simulink model "spring_mass"  (R2021b)
settings: Solver=VariableStepAuto  StartTime=0.0  StopTime=10.0  RelTol=1e-3
settings Model: Creator=cgrundm  LastModifiedBy=cgrundm

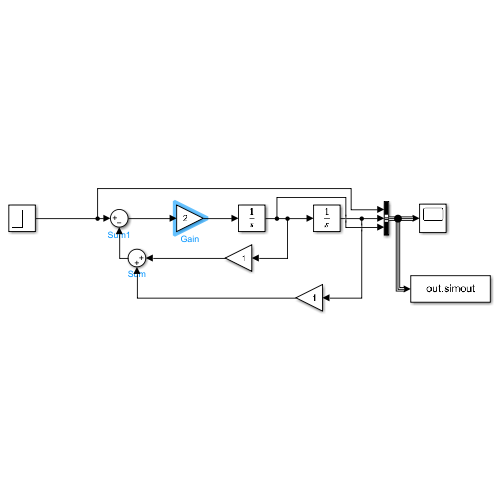
[thumbnail: Simulink's stored preview of the top-level diagram]
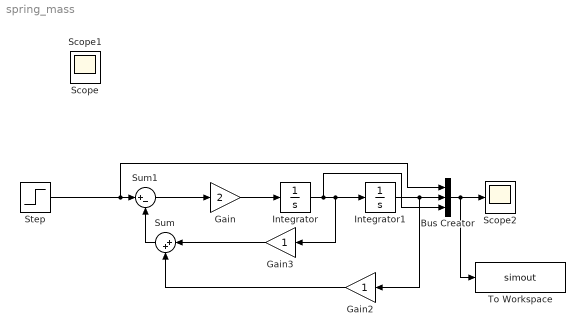
== system spring_mass ==
  Bus Creator : BusCreator  Inputs=3
  Gain : Gain  Gain=2
  Gain2 : Gain
  Gain3 : Gain
  Integrator : Integrator
  Integrator1 : Integrator
  Scope2 : Scope
  Step : Step  SampleTime=0
  Sum : Sum  Inputs=|++
  Sum1 : Sum  Inputs=|+-
  To Workspace : ToWorkspace  VariableName=simout  SaveFormat=Timeseries  SampleTime=-1
  Scope : Scope
  Scope1 : Scope
  wires:
  Integrator1/1 -> Gain2/1, Bus Creator/2
  Integrator/1 -> Bus Creator/3, Gain3/1, Integrator1/1
  Gain3/1 -> Sum/1
  Gain2/1 -> Sum/2
  Step/1 -> Bus Creator/1, Sum1/1
  Sum/1 -> Sum1/2
  Sum1/1 -> Gain/1
  Gain/1 -> Integrator/1
  Bus Creator/1 -> To Workspace/1, Scope2/1
